simulink library "rsc"  (Simulink 8.1)
settings: Solver=ode1  StartTime=0.0  StopTime=Inf  FixedStep=0.001  RelTol=1e-3
PostLoadFcn:
  | , if any(exist('dsrtsu_mdlpostloadfcn', 'file') == [2, 3, 6]), try dsrtsu_mdlpostloadfcn('Execute', bdroot); catch fprintf('Error in PostLoadFcn (dsrtsu_mdlpostloadfcn) for model "%s":\n %s\n', bdroot, lasterr); end, end,
undefined symbols (not defined in the file or in its folder): FALSE, KJUD_ACCGapErrorGParam_num, KJUD_ACCGapFFParam_num, KJUD_ACCGapInitialIParam_num, KJUD_ACCGapKiParam_num, KJUD_ACCGapKpParam_num, KJUD_ACCGapMaxIParam_num, KJUD_ACCGapMinIParam_num, KJUD_ACCGapResetIParam_num
libraries: hcu_lib x1
settings Model: DSRTSU_INTERNAL_RTI_VER=450  DSRTSU_INTERNAL_RTI_TYPE=rti1401  RTICANMMDATA=struct('GeneralSetupData',struct('modelroot','D:\Projects\ELN150201\Repositories\Internal\Phase3\branches\ACC_Test_Tracks\AdasDragon\software\sw_development\arch\app\jud','generalsettings',struct('filesettings',struct('destfolder',struct('Name','RTICANMM_FILES','Check',1),'buildfolder',struct('Name','.','Check',1),'AbsDestfolder',struct('Name','D:\Projects\ELN150201\Repositories\Internal\Phase3\branches\ACC_Test_Tracks\AdasDragon\software\sw_development\arch\app\jud\RTICANMM_FILES'),'AbsBuildfolder',struct('Name','D:\Projects\ELN150201\Repositories\Internal\Phase3\branches\ACC_Test_Tracks\AdasDragon\software\sw_development\arch\app\jud'))),'options',struct('addpaths',1,'rmpaths',1,'addtrcexclusion',logical(1),'cannavigator',struct('checkmonitoring',0),'show_usrtrc',0,'use_usrtrc',0),'advanced',struct('options',[1 1 1 1 1 1 1 1 1 1 1 1 1 1 1 1 1 1 1 1 1 1 1 1 1 1 1 1 1 1 1 1 1 1 1 1 1 1 1 1 1 1 1 1 1 1 1 1 1 1 1 1 1 1 1 1 1 1 1 1 1 1 1 1 1 1 1 1 1 1 1 1 1 1 1 1 1 1 1 1 1 1 1 1 1 1 1 1 1 1 1 1 1 1 1 1 1 1 1 1]),'MPSetup',{{}},'modelname','rsc','block','rsc'))  DSRTSU_INTERNAL_RTIFPGA=40  Creator=tescamilla  LastModifiedBy=AT015086

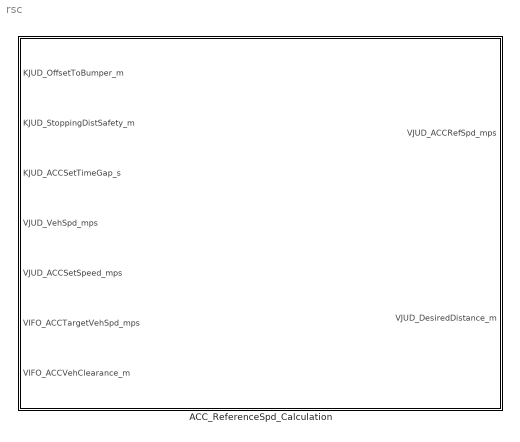
== system rsc ==
  ACC_ReferenceSpd_Calculation : Subsystem

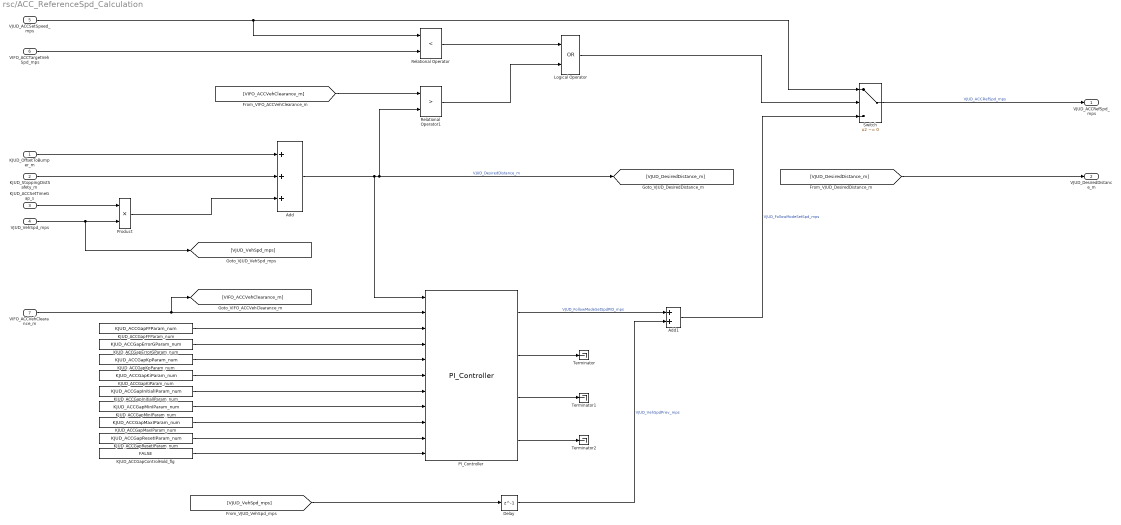
== system rsc/ACC_ReferenceSpd_Calculation ==
  KJUD_OffsetToBumper_m : Inport
  KJUD_StoppingDistSafety_m : Inport  Port=2
  KJUD_ACCSetTimeGap_s : Inport  Port=3
  VJUD_VehSpd_mps : Inport  Port=4
  VJUD_ACCSetSpeed_mps : Inport  Port=5
  VIFO_ACCTargetVehSpd_mps : Inport  Port=6
  VIFO_ACCVehClearance_m : Inport  Port=7
  Add : Sum  Inputs=+++  SaturateOnIntegerOverflow=off  InputSameDT=off  OutDataTypeStr=Inherit: Inherit via internal rule
  Add1 : Sum  SaturateOnIntegerOverflow=off  InputSameDT=off  OutDataTypeStr=Inherit: Inherit via internal rule
  Delay : Delay  DelayLength=1  InitialCondition=0
  KJUD_ACCGapControlHold_flg : Constant  Value=FALSE  OutDataTypeStr=boolean
  KJUD_ACCGapErrorGParam_num : Constant  Value=KJUD_ACCGapErrorGParam_num
  KJUD_ACCGapFFParam_num : Constant  Value=KJUD_ACCGapFFParam_num
  KJUD_ACCGapInitialIParam_num : Constant  Value=KJUD_ACCGapInitialIParam_num
  KJUD_ACCGapKiParam_num : Constant  Value=KJUD_ACCGapKiParam_num
  KJUD_ACCGapKpParam_num : Constant  Value=KJUD_ACCGapKpParam_num
  KJUD_ACCGapMaxIParam_num : Constant  Value=KJUD_ACCGapMaxIParam_num
  KJUD_ACCGapMinIParam_num : Constant  Value=KJUD_ACCGapMinIParam_num
  KJUD_ACCGapResetIParam_num : Constant  Value=KJUD_ACCGapResetIParam_num
  Logical Operator : Logic  Operator=OR  AllPortsSameDT=off  OutDataTypeStr=boolean
  PI_Controller : hcu_lib/PI_Controller  SystemSampleTime=-1
  Product : Product  SaturateOnIntegerOverflow=off  RndMeth=Floor  InputSameDT=off  OutDataTypeStr=Inherit: Inherit via internal rule
  Relational Operator : RelationalOperator  Operator=<  OutDataTypeStr=boolean  InputSameDT=off
  Relational Operator1 : RelationalOperator  Operator=>  OutDataTypeStr=boolean  InputSameDT=off
  Switch : Switch  Criteria=u2 ~= 0  SaturateOnIntegerOverflow=off  InputSameDT=off
  Terminator : Terminator
  Terminator1 : Terminator
  Terminator2 : Terminator
  VJUD_ACCRefSpd_mps : Outport
  VJUD_DesiredDistance_m : Outport  Port=2
  wires:
  Delay/1 -> Add1/2  "VJUD_VehSpdPrev_mps"
  [VJUD_VehSpd_mps] -> Delay/1
  PI_Controller/1 -> Add1/1  "VJUD_FollowModeSetSpdPID_mps"
  [VJUD_DesiredDistance_m] -> VJUD_DesiredDistance_m/1
  PI_Controller/4 -> Terminator2/1
  PI_Controller/2 -> Terminator/1
  PI_Controller/3 -> Terminator1/1
  Relational Operator1/1 -> Logical Operator/2
  [VIFO_ACCVehClearance_m] -> Relational Operator1/1
  KJUD_ACCGapKiParam_num/1 -> PI_Controller/6
  KJUD_ACCGapErrorGParam_num/1 -> PI_Controller/4
  KJUD_ACCGapControlHold_flg/1 -> PI_Controller/11
  KJUD_ACCGapKpParam_num/1 -> PI_Controller/5
  KJUD_ACCGapFFParam_num/1 -> PI_Controller/3
  KJUD_ACCGapMinIParam_num/1 -> PI_Controller/8
  KJUD_ACCGapResetIParam_num/1 -> PI_Controller/10
  KJUD_ACCGapMaxIParam_num/1 -> PI_Controller/9
  KJUD_ACCGapInitialIParam_num/1 -> PI_Controller/7
  Add1/1 -> Switch/3  "VJUD_FollowModeSetSpd_mps"
  Add/1 -> PI_Controller/1, Relational Operator1/2, [VJUD_DesiredDistance_m]  "VJUD_DesiredDistance_m"
  VIFO_ACCVehClearance_m/1 -> PI_Controller/2, [VIFO_ACCVehClearance_m]
  Relational Operator/1 -> Logical Operator/1
  VIFO_ACCTargetVehSpd_mps/1 -> Relational Operator/2
  Logical Operator/1 -> Switch/2
  KJUD_ACCSetTimeGap_s/1 -> Product/1
  VJUD_VehSpd_mps/1 -> Product/2, [VJUD_VehSpd_mps]
  VJUD_ACCSetSpeed_mps/1 -> Switch/1, Relational Operator/1
  KJUD_StoppingDistSafety_m/1 -> Add/2
  Switch/1 -> VJUD_ACCRefSpd_mps/1  "VJUD_ACCRefSpd_mps"
  Product/1 -> Add/3
  KJUD_OffsetToBumper_m/1 -> Add/1
